simulink model "SS_task6_5_2020"  (R2021a)
settings: Solver=FixedStepAuto  StartTime=0.0  StopTime=20  FixedStep=0.01  RelTol=1e-3
values from neighbouring files (symbols this model uses):
  A_cl = [ 0 1 0 0 ... (first row only)    [Copy_of_Lab_3_ale.m]    (also in Lab_3_ale.m; mass_2dof.m)
  A_ss = [ 0 1 0 0 ... (first row only)    [Copy_of_Lab_3_ale.m]    (also in Lab_3_ale.m; mass_2dof.m)
  B_cl = [ 0 0 ... (first row only)    [Copy_of_Lab_3_ale.m]    (also in Lab_3_ale.m; mass_2dof.m)
  B_ss = [0 0 0 ... (first row only)    [Copy_of_Lab_3_ale.m]    (also in Lab_3_ale.m; mass_2dof.m)
  C_cl = [1 0 0 0]    [Copy_of_Lab_3_ale.m]    (also in Lab_3_ale.m; mass_2dof.m)
  C_ss = [1 0 0 0]    [Copy_of_Lab_3_ale.m]    (also in Lab_3_ale.m; mass_2dof.m)
  D_cl = [0 0]    [Copy_of_Lab_3_ale.m]    (also in Lab_3_ale.m; mass_2dof.m)
  D_ss = [0 0 0]    [Copy_of_Lab_3_ale.m]    (also in Lab_3_ale.m; mass_2dof.m)
  T = 1.5    [Copy_of_Lab_3_ale.m]    (also in Lab_3_ale.m; mass_2dof.m = 0.12)
  wn = wn_und_1dof    [Copy_of_Lab_3_ale.m]    (also in H_inf_ctrl_11_2.m = eig(Ask); H_inf_ctrl_11_2_m.m = eig(Ask); Lab_3_ale.m = sqrt(kp/mp); mass_2dof.m)
undefined symbols (not defined in the file or in its folder): sigbuilder_block
settings Model: Creator=rivaa  LastModifiedBy=rivaa

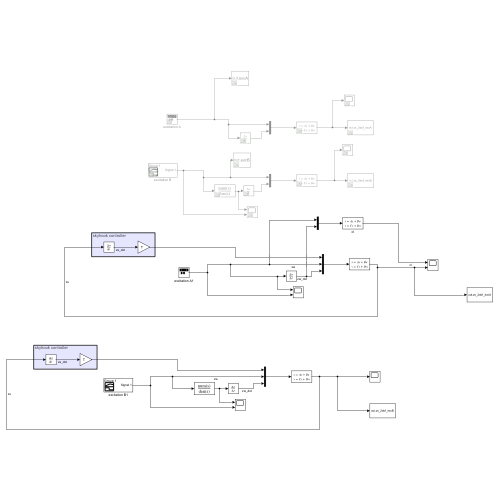
[thumbnail: Simulink's stored preview of the top-level diagram]
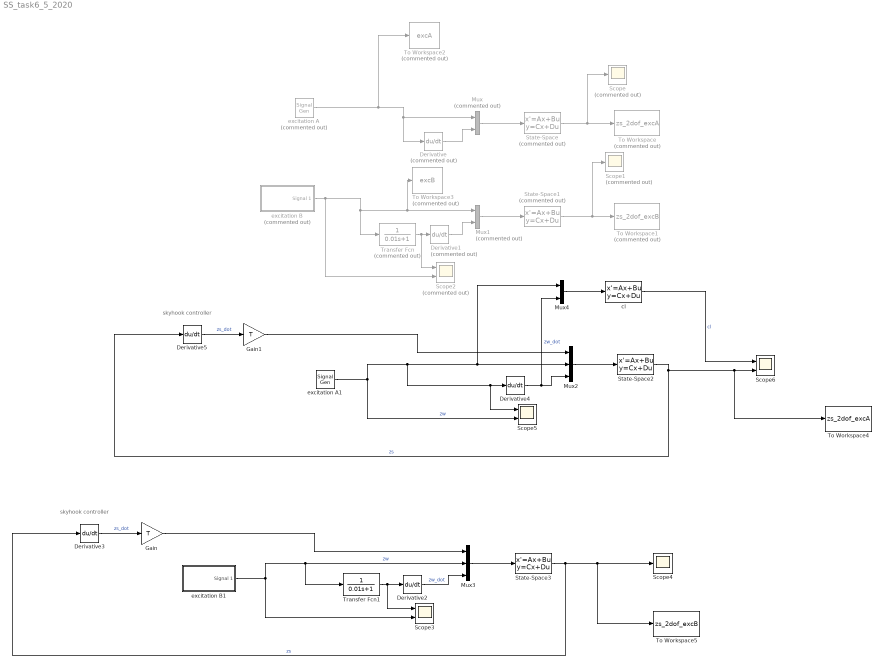
== system SS_task6_5_2020 ==
  note: skyhook controller
  note: skyhook controller
  Derivative : Derivative  Commented=on
  Derivative1 : Derivative  Commented=on
  Derivative{2..5} (4 alike) : Derivative
  Gain : Gain  Gain=T
  Gain1 : Gain  Gain=T
  Mux : Mux  Commented=on  Inputs=2
  Mux1 : Mux  Commented=on  Inputs=2
  Mux2 : Mux  Inputs=3
  Mux3 : Mux  Inputs=3
  Mux4 : Mux  Inputs=2
  Scope : Scope  Commented=on
  Scope1 : Scope  Commented=on
  Scope2 : Scope  Commented=on  NumInputPorts=2
  Scope3 : Scope  NumInputPorts=2
  Scope4 : Scope
  Scope5 : Scope  NumInputPorts=2
  Scope6 : Scope  NumInputPorts=2
  State-Space : StateSpace  Commented=on  A=A_ss  B=B_ss  C=C_ss  D=D_ss  InitialCondition=0
  State-Space1 : StateSpace  Commented=on  A=A_ss  B=B_ss  C=C_ss  D=D_ss  InitialCondition=0
  State-Space2 : StateSpace  A=A_ss  B=B_ss  C=C_ss  D=D_ss  InitialCondition=0
  State-Space3 : StateSpace  A=A_ss  B=B_ss  C=C_ss  D=D_ss  InitialCondition=0
  To Workspace : ToWorkspace  Commented=on  VariableName=zs_2dof_excA  SampleTime=-1
      settings: Save2DSignal=2-D array (concatenate along first dimension)
  To Workspace1 : ToWorkspace  Commented=on  VariableName=zs_2dof_excB  SampleTime=-1
      settings: Save2DSignal=2-D array (concatenate along first dimension)
  To Workspace2 : ToWorkspace  Commented=on  VariableName=excA  SampleTime=-1
      settings: Save2DSignal=2-D array (concatenate along first dimension)
  To Workspace3 : ToWorkspace  Commented=on  VariableName=excB  SampleTime=-1
      settings: Save2DSignal=2-D array (concatenate along first dimension)
  To Workspace4 : ToWorkspace  VariableName=zs_2dof_excA  SampleTime=-1
      settings: Save2DSignal=2-D array (concatenate along first dimension)
  To Workspace5 : ToWorkspace  VariableName=zs_2dof_excB  SampleTime=-1
      settings: Save2DSignal=2-D array (concatenate along first dimension)
  Transfer Fcn : TransferFcn  Commented=on  Denominator=[0.01 1]
  Transfer Fcn1 : TransferFcn  Denominator=[0.01 1]
  cl : StateSpace  A=A_cl  B=B_cl  C=C_cl  D=D_cl  InitialCondition=0
  excitation A : SignalGenerator  Commented=on  Amplitude=0.05  Frequency=wn  Units=rad/sec
  excitation A1 : SignalGenerator  Amplitude=0.05  Frequency=wn  Units=rad/sec
  excitation B : Subsystem  Tag=STV Subsys  Commented=on  LoadFcn=sigbuilder_block('load');  StartFcn=sigbuilder_block('start');  StopFcn=sigbuilder_block('stop');  ClipboardFcn=sigbuilder_block('clipboard');  mask(Sigbuilder block){tuvar=[0:10]}
      mask help: Simulink:masks:SigbuilderBlock_MD
      mask init:
      | if ~strcmp(get_param(bdroot(gcbh),'SimulationStatus'),'stopped') tuvar = sigbuilder_block('maskInit'); end
      settings: CopyFcn=sigbuilder_block('copy');  DeleteFcn=sigbuilder_block('delete');  ModelCloseFcn=sigbuilder_block('modelClose');  PreSaveFcn=sigbuilder_block('preSave');  PauseFcn=sigbuilder_block('pause');  ContinueFcn=sigbuilder_block('continue');  NameChangeFcn=sigbuilder_block('namechange');  OpenFcn=sigbuilder_block('open',[437.6 199.2 550.4 400 ]);  CloseFcn=sigbuilder_block('close');
      mask Display: plot(0, 0, 100, 100,[2, 2, 32, 32, 2], [68, 8, 8, 68, 68],[32, 2], [38, 38], [32, 19, 2],[53, 60, 44], [32, 17, 17, 2],[16, 16, 31, 31]);txt = getActiveGroup(gcbh);text(2, 100, txt,'verticalAlignment', 'top');
  excitation B1 : Subsystem  Tag=STV Subsys  LoadFcn=sigbuilder_block('load');  StartFcn=sigbuilder_block('start');  StopFcn=sigbuilder_block('stop');  ClipboardFcn=sigbuilder_block('clipboard');  mask(Sigbuilder block){tuvar=[0:10]}
      mask help: Simulink:masks:SigbuilderBlock_MD
      mask init:
      | if ~strcmp(get_param(bdroot(gcbh),'SimulationStatus'),'stopped') tuvar = sigbuilder_block('maskInit'); end
      settings: CopyFcn=sigbuilder_block('copy');  DeleteFcn=sigbuilder_block('delete');  ModelCloseFcn=sigbuilder_block('modelClose');  PreSaveFcn=sigbuilder_block('preSave');  PauseFcn=sigbuilder_block('pause');  ContinueFcn=sigbuilder_block('continue');  NameChangeFcn=sigbuilder_block('namechange');  OpenFcn=sigbuilder_block('open',[437.6 199.2 550.4 400 ]);  CloseFcn=sigbuilder_block('close');
      mask Display: plot(0, 0, 100, 100,[2, 2, 32, 32, 2], [68, 8, 8, 68, 68],[32, 2], [38, 38], [32, 19, 2],[53, 60, 44], [32, 17, 17, 2],[16, 16, 31, 31]);txt = getActiveGroup(gcbh);text(2, 100, txt,'verticalAlignment', 'top');
  wires:
  State-Space/1 -> Scope/1, To Workspace/1
  excitation A/1 -> To Workspace2/1, Derivative/1, Mux/1
  Derivative/1 -> Mux/2
  Mux/1 -> State-Space/1
  Mux1/1 -> State-Space1/1
  Derivative1/1 -> Mux1/2
  excitation B/1(Signal 1) -> Scope2/2, To Workspace3/1, Mux1/1, Transfer Fcn/1
  State-Space1/1 -> Scope1/1, To Workspace1/1
  Transfer Fcn/1 -> Scope2/1, Derivative1/1
  Mux3/1 -> State-Space3/1
  Transfer Fcn1/1 -> Scope3/1, Derivative2/1
  excitation B1/1(Signal 1) -> Scope3/2, Transfer Fcn1/1, Mux3/2  "zw"
  Derivative2/1 -> Mux3/3  "zw_dot"
  State-Space3/1 -> To Workspace5/1, Scope4/1, Derivative3/1  "zs"
  Derivative3/1 -> Gain/1  "zs_dot"
  Gain/1 -> Mux3/1
  Gain1/1 -> Mux2/1
  Derivative5/1 -> Gain1/1  "zs_dot"
  State-Space2/1 -> Derivative5/1, To Workspace4/1, Scope6/2  "zs"
  Derivative4/1 -> Mux4/2, Mux2/3  "zw_dot"
  excitation A1/1 -> Derivative4/1, Scope5/1, Mux4/1, Mux2/2, Scope5/2  "zw"
  Mux2/1 -> State-Space2/1
  Mux4/1 -> cl/1
  cl/1 -> Scope6/1  "cl"

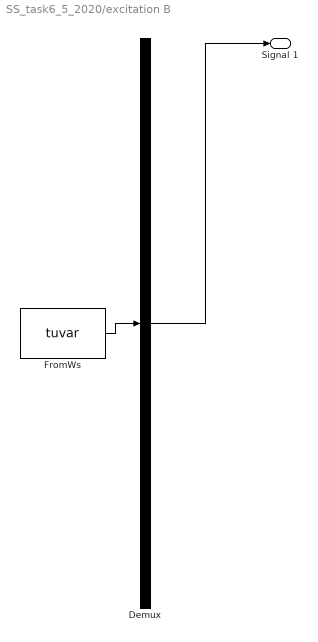
== system SS_task6_5_2020/excitation B ==
  Demux : Demux  Tag=STV Demux  Outputs=1
      settings: DisplayOption=none
  FromWs : FromWorkspace  Tag=STV FromWs  VariableName=tuvar
      SigBuilderData=|
      | common.afterFinalStr = 'Extrapolate'
      | common.sampleTime = 0
      | dataSet.timeRange = [0 10]
      | dataSet.name = 'Group 1'
      | sbobj.Groups.Name = 'Group 1'
      | sbobj.Groups.Signals.Name = 'Signal 1'
      | sbobj.Groups.Signals.XData = [0 4 4 4.1 4.1 10]
      | sbobj.Groups.Signals.YData = [0 0 0.05 0.05 0 0]
  Signal 1 : Outport  Tag=STV Outport
  wires:
  Demux/1 -> Signal 1/1
  FromWs/1 -> Demux/1

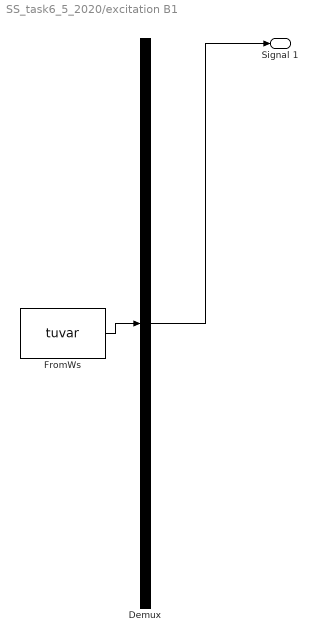
== system SS_task6_5_2020/excitation B1 ==
  Demux : Demux  Tag=STV Demux  Outputs=1
      settings: DisplayOption=none
  FromWs : FromWorkspace  Tag=STV FromWs  VariableName=tuvar
      SigBuilderData=|
      | common.afterFinalStr = 'Extrapolate'
      | common.sampleTime = 0
      | dataSet.timeRange = [0 10]
      | dataSet.name = 'Group 1'
      | sbobj.Groups.Name = 'Group 1'
      | sbobj.Groups.Signals.Name = 'Signal 1'
      | sbobj.Groups.Signals.XData = [0 4 4 4.1 4.1 10]
      | sbobj.Groups.Signals.YData = [0 0 0.05 0.05 0 0]
  Signal 1 : Outport  Tag=STV Outport
  wires:
  FromWs/1 -> Demux/1
  Demux/1 -> Signal 1/1
